simulink model "create_turn_vehicle_ref"  (R2024b)
settings: Solver=FixedStepAuto  StartTime=0.0  StopTime=end_time_vehicle  FixedStep=0.02  RelTol=1e-3
libraries: SignalEditorBlockLib x1
settings Model: Creator=tshintai  LastModifiedBy=tshintai
settings SolverCC: AlgebraicLoopSolver=TrustRegion
settings DataIOCC: SignalLogging=off  DSMLogging=off  SaveTime=off  ReturnWorkspaceOutputsName=turn_vehicle_ref_data
settings OptimizationCC: ReuseModelBlockBuffer=off
settings DebuggingCC: UnconnectedInputMsg=warning  UnconnectedOutputMsg=warning  UnconnectedLineMsg=warning
settings ModelReferenceCC: EnableRefExpFcnMdlSchedulingChecks=on
settings RTWCC: GPUComputeCapability=3.5  DLArmComputeVersion=19.05

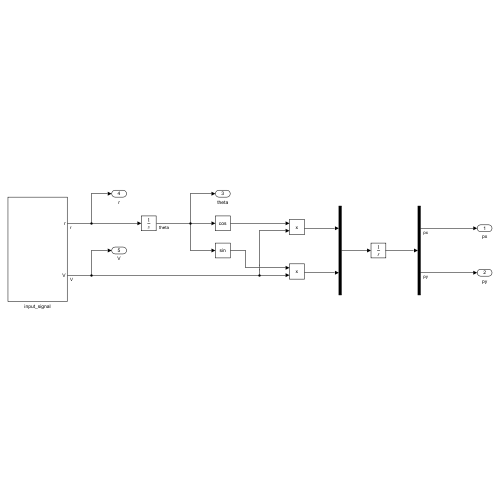
[thumbnail: Simulink's stored preview of the top-level diagram]
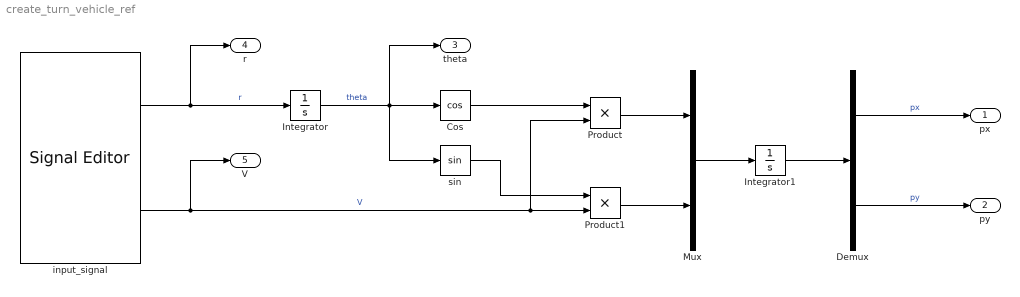
== system create_turn_vehicle_ref ==
  Cos : Trigonometry  Operator=cos
  Demux : Demux  Outputs=2
  Integrator : Integrator
  Integrator1 : Integrator
  Mux : Mux  Inputs=2
  Product : Product
  Product1 : Product
  input_signal : SignalEditorBlockLib/Signal Editor  FileName=ref_elements_signal.mat  ActiveScenario=elements_of_regular_circle_vehicle  ActiveSignal=r  IsBus=off  OutputBusObjectStr=Bus: BusObject  SampleTime=0  ZeroCross=off  OutputAfterFinalValue=Holding final value  Unit=inherit  PreserveSignalName=on  ApplySigPropsToAllScenarios=on  ApplySigPropsToAllSignals=off
  sin : Trigonometry
  px : Outport
  py : Outport  Port=2
  theta : Outport  Port=3
  r : Outport  Port=4
  V : Outport  Port=5
  wires:
  input_signal/1 -> r/1, Integrator/1  "r"
  Integrator/1 -> theta/1, sin/1, Cos/1  "theta"
  Cos/1 -> Product/1
  input_signal/2 -> V/1, Product/2, Product1/2  "V"
  sin/1 -> Product1/1
  Product/1 -> Mux/1
  Product1/1 -> Mux/2
  Mux/1 -> Integrator1/1
  Integrator1/1 -> Demux/1
  Demux/1 -> px/1  "px"
  Demux/2 -> py/1  "py"
